simulink model "lstmpi_project"  (R2025a)
settings: Solver=ode4  StartTime=0.0  StopTime=1  FixedStep=0.001  RelTol=1e-3
settings Model: Creator=aswin  LastModifiedBy=hrish

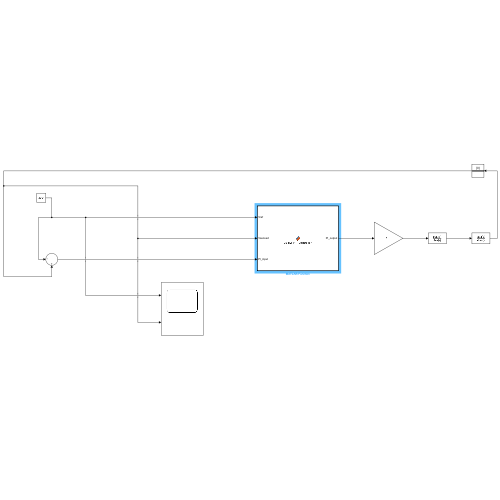
[thumbnail: Simulink's stored preview of the top-level diagram]
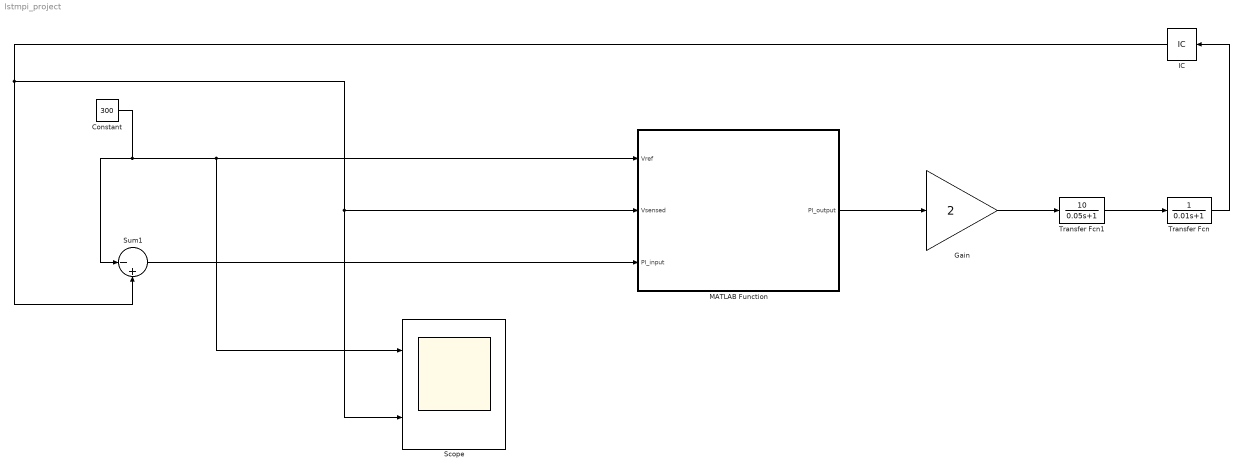
== system lstmpi_project ==
  Constant : Constant  Value=300
  Gain : Gain  Gain=2
  IC : InitialCondition  Value=0
  MATLAB Function : MATLAB Function  TreatAsAtomicUnit=on  SystemSampleTime=0.001
  Scope : Scope  NumInputPorts=2
      settings: ActiveDisplayYMinimum=200  ActiveDisplayYMaximum=400
  Sum1 : Sum  Inputs=|-+
  Transfer Fcn : TransferFcn  Denominator=[0.01 1]
  Transfer Fcn1 : TransferFcn  Numerator=[10]  Denominator=[0.05 1]
  wires:
  Constant/1 -> Scope/1, MATLAB Function/1(Vref), Sum1/1
  Sum1/1 -> MATLAB Function/3(PI_input)
  MATLAB Function/1(PI_output) -> Gain/1
  Gain/1 -> Transfer Fcn1/1
  Transfer Fcn1/1 -> Transfer Fcn/1
  Transfer Fcn/1 -> IC/1
  IC/1 -> Sum1/2, Scope/2, MATLAB Function/2(Vsensed)

== matlab function lstmpi_project/MATLAB Function ==
  data: Vref input; PI_output output; Vsensed input; PI_input input
function PI_output = LSTM_PI_Controller(Vref, Vsensed, PI_input)

persistent weights scalers
persistent seq_buffer
persistent PI_input_lag1 PI_input_lag2 PI_out_lag1
persistent error_cumsum
persistent step_count

if isempty(weights)
    raw_w = load('model_weights_full.mat');
    raw_s = load('scaler_params (2).mat');
    
    % Cast ALL weight matrices to double
    weights.Wf1 = double(raw_w.Wf1); weights.Uf1 = double(raw_w.Uf1); weights.Bf1 = double(raw_w.Bf1);
    weights.Wb1 = double(raw_w.Wb1); weights.Ub1 = double(raw_w.Ub1); weights.Bb1 = double(raw_w.Bb1);
    weights.Wf2 = double(raw_w.Wf2); weights.Uf2 = double(raw_w.Uf2); weights.Bf2 = double(raw_w.Bf2);
    weights.Wb2 = double(raw_w.Wb2); weights.Ub2 = double(raw_w.Ub2); weights.Bb2 = double(raw_w.Bb2);
    weights.W3  = double(raw_w.W3);  weights.U3  = double(raw_w.U3);  weights.B3  = double(raw_w.B3);
    weights.Wd1 = double(raw_w.Wd1); weights.Bd1 = double(raw_w.Bd1);
    weights.Wd2 = double(raw_w.Wd2); weights.Bd2 = double(raw_w.Bd2);
    
    % Cast scaler params to double
    scalers.X_min = double(raw_s.X_min);
    scalers.X_max = double(raw_s.X_max);
    scalers.y_min = double(raw_s.y_min);
    scalers.y_max = double(raw_s.y_max);
    
    seq_buffer    = zeros(60, 9);   % double by default
    PI_input_lag1 = 0;
    PI_input_lag2 = 0;
    PI_out_lag1   = 0;
    error_cumsum  = 0;
    step_count    = 0;
end

%Feature engineering
Error        = double(Vref) - double(Vsensed);
Error_diff   = Error - (PI_input_lag1 - PI_input_lag2);
error_cumsum = error_cumsum + Error;

x_raw = [double(Vref), double(Vsensed), double(PI_input), Error, ...
         PI_input_lag1, PI_input_lag2, PI_out_lag1, ...
         Error_diff, error_cumsum];

%MinMax scaling
denom = scalers.X_max - scalers.X_min;
denom(denom == 0) = 1;
x_scaled = (x_raw - scalers.X_min) ./ denom;

%Rolling buffer
seq_buffer = [seq_buffer(2:end, :); x_scaled];
step_count = step_count + 1;

%Forward pass
if step_count < 60
    PI_output = 0;
else
    H1 = bilstm_layer(seq_buffer, weights.Wf1, weights.Uf1, weights.Bf1, weights.Wb1, weights.Ub1, weights.Bb1, 256);
    H2 = bilstm_layer(H1,         weights.Wf2, weights.Uf2, weights.Bf2, weights.Wb2, weights.Ub2, weights.Bb2, 128);
    h3 = lstm_last(H2, weights.W3, weights.U3, weights.B3, 64);
    d1 = max(0, h3 * weights.Wd1 + weights.Bd1);
    y_scaled  = d1 * weights.Wd2 + weights.Bd2;
    PI_output = double(y_scaled * (scalers.y_max - scalers.y_min) + scalers.y_min);
end

%Update lag memory
PI_input_lag2 = PI_input_lag1;
PI_input_lag1 = double(PI_input);
PI_out_lag1   = PI_output;

end

% ── Bidirectional LSTM ────────────────────────────────────────────────────────
function H = bilstm_layer(X, Wf, Uf, Bf, Wb, Ub, Bb, H_size)
    T  = size(X, 1);
    Hf = zeros(T, H_size);   % double
    Hb = zeros(T, H_size);   % double
    hf = zeros(1, H_size);   cf = zeros(1, H_size);
    hb = zeros(1, H_size);   cb = zeros(1, H_size);
    for t = 1:T
        [hf, cf] = lstm_step(X(t,:), hf, cf, Wf, Uf, Bf, H_size);
        Hf(t,:)  = hf;
    end
    for t = T:-1:1
        [hb, cb] = lstm_step(X(t,:), hb, cb, Wb, Ub, Bb, H_size);
        Hb(t,:)  = hb;
    end
    H = [Hf, Hb];
end

% ── LSTM last timestep only ───────────────────────────────────────────────────
function h = lstm_last(X, W, U, B, H_size)
    T = size(X, 1);
    h = zeros(1, H_size);
    c = zeros(1, H_size);
    for t = 1:T
        [h, c] = lstm_step(X(t,:), h, c, W, U, B, H_size);
    end
end

% ── Single LSTM step ──────────────────────────────────────────────────────────
function [h_new, c_new] = lstm_step(x, h, c, W, U, B, H_size)
    gates = x * W  +  h * U  +  B;
    i_g = sigmoid_fn( gates(1          : H_size)   );
    f_g = sigmoid_fn( gates(H_size+1   : 2*H_size) );
    g_g = tanh(       gates(2*H_size+1 : 3*H_size) );
    o_g = sigmoid_fn( gates(3*H_size+1 : 4*H_size) );
    c_new = f_g .* c  +  i_g .* g_g;
    h_new = o_g .* tanh(c_new);
end

% ── Sigmoid ───────────────────────────────────────────────────────────────────
function y = sigmoid_fn(x)
    y = 1 ./ (1 + exp(-x));
end
